simulink model "THIPWM_Three_Phase_Two_Level_Inverter"  (R2022a)
settings: Solver=ode4  StartTime=0.0  StopTime=1  FixedStep=1e-5  RelTol=1e-3
libraries: spsIGBTLib x6, spsSeriesRLCBranchLib x3, spsDCVoltageSourceLib x1, spsGroundLib x1, spsSawtoothGeneratorLib x1, spsThreePhaseVIMeasurementLib x1, spspowerguiLib x1
settings Model: Creator=nikos  LastModifiedBy=nikos

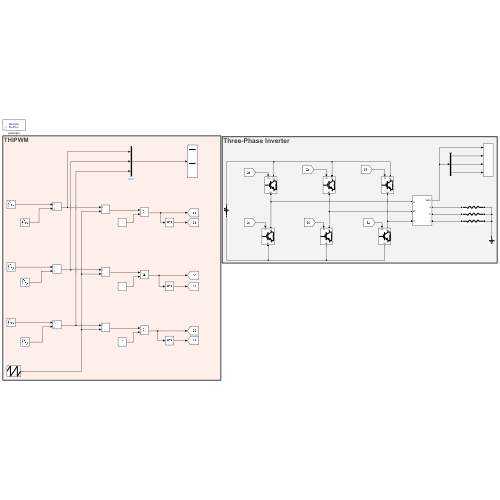
[thumbnail: Simulink's stored preview of the top-level diagram]
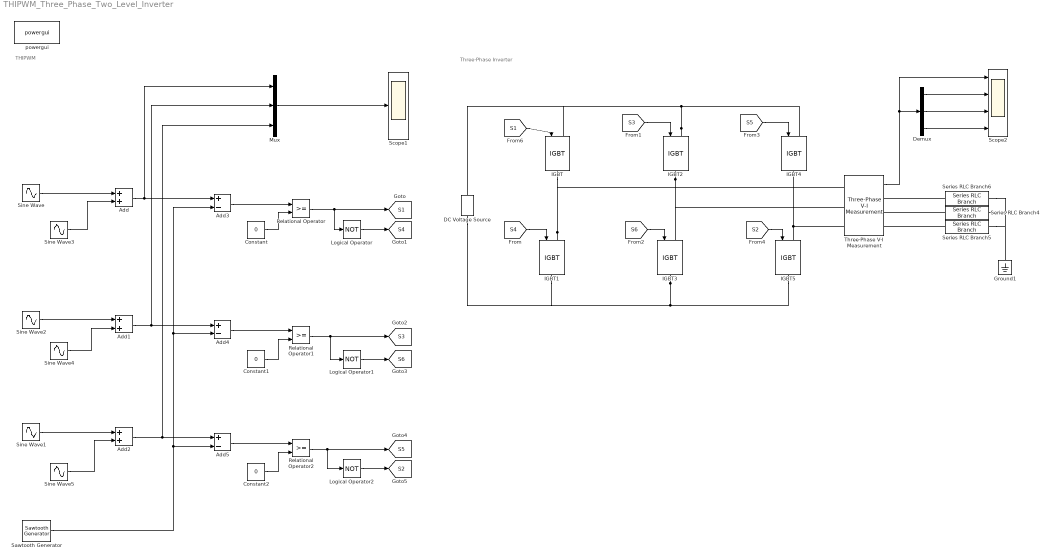
== system THIPWM_Three_Phase_Two_Level_Inverter ==
  note: THIPWM
  note: Three-Phase Inverter
  Add : Sum
  Add1 : Sum
  Add2 : Sum
  Add3 : Sum  Inputs=+-
  Add4 : Sum  Inputs=+-
  Add5 : Sum  Inputs=+-
  Constant : Constant  Value=0
  Constant1 : Constant  Value=0
  Constant2 : Constant  Value=0
  DC Voltage Source : spsDCVoltageSourceLib/DC Voltage Source  Amplitude=400  Measurements=None
  Demux : Demux  Outputs=3
  Ground1 : spsGroundLib/Ground  LConnTagsString=a
  IGBT{,1..5} (6 alike) : spsIGBTLib/IGBT  Ron=0.001  Lon=0  Vf=1  Tf=1e-6  Tt=2e-6  IC=0  Rs=1e5  Cs=inf  Measurements=off
  Logical Operator : Logic  Operator=NOT  AllPortsSameDT=off  OutDataTypeStr=boolean
  Logical Operator1 : Logic  Operator=NOT  AllPortsSameDT=off  OutDataTypeStr=boolean
  Logical Operator2 : Logic  Operator=NOT  AllPortsSameDT=off  OutDataTypeStr=boolean
  Mux : Mux  Inputs=3
  Relational Operator : RelationalOperator  OutDataTypeStr=boolean  RndMeth=Simplest  InputSameDT=off
  Relational Operator1 : RelationalOperator  OutDataTypeStr=boolean  RndMeth=Simplest  InputSameDT=off
  Relational Operator2 : RelationalOperator  OutDataTypeStr=boolean  RndMeth=Simplest  InputSameDT=off
  Sawtooth Generator : spsSawtoothGeneratorLib/Sawtooth Generator  Freq=2e3  Phase=180  Ts=0
  Scope1 : Scope
  Scope2 : Scope  NumInputPorts=4
  Series RLC Branch4 : spsSeriesRLCBranchLib/Series RLC Branch  LConnTagsString=__new0  RConnTagsString=__new0  BranchType=R  Resistance=100  Inductance=1e-3  SetiL0=off  InitialCurrent=0  Capacitance=1e-6  Setx0=off  InitialVoltage=0  Measurements=None
  Series RLC Branch5 : spsSeriesRLCBranchLib/Series RLC Branch  LConnTagsString=__new0  RConnTagsString=__new0  BranchType=R  Resistance=100  Inductance=1e-3  SetiL0=off  InitialCurrent=0  Capacitance=1e-6  Setx0=off  InitialVoltage=0  Measurements=None
  Series RLC Branch6 : spsSeriesRLCBranchLib/Series RLC Branch  LConnTagsString=__new0  RConnTagsString=__new0  BranchType=R  Resistance=100  Inductance=1e-3  SetiL0=off  InitialCurrent=0  Capacitance=1e-6  Setx0=off  InitialVoltage=0  Measurements=None
  Sine Wave : Sin  Amplitude=1.1547  Frequency=2*pi*50  SampleTime=0
  Sine Wave1 : Sin  Amplitude=1.1547  Frequency=2*pi*50  Phase=4*pi/3  SampleTime=0
  Sine Wave2 : Sin  Amplitude=1.1547  Frequency=2*pi*50  Phase=2*pi/3  SampleTime=0
  Sine Wave3 : Sin  Amplitude=0.193  Frequency=2*pi*50*3  SampleTime=0
  Sine Wave4 : Sin  Amplitude=0.193  Frequency=2*pi*50*3  SampleTime=0
  Sine Wave5 : Sin  Amplitude=0.193  Frequency=2*pi*50*3  SampleTime=0
  Three-Phase V-I Measurement : spsThreePhaseVIMeasurementLib/Three-Phase V-I Measurement  VoltageMeasurement=phase-to-ground  SetLabelV=off  LabelV=Vabc  Vpu=off  VpuLL=off  CurrentMeasurement=no  SetLabelI=off  LabelI=Iabc  Ipu=off  Pbase=100e6  Vbase=500e3  OutputType=Complex  PhasorSimulation=off  PSBequivalent=0
  powergui : spspowerguiLib/powergui  Priority=1  SimulationMode=Discrete  SampleTime=50e-6  frequency=60  Iterations=50  frequencyindice=0  Pbase=100e6  ErrMax=1e-4  UnitsV=kV  UnitsW=MW  buscounter=0  FunctionMessages=off  echomessages=off  EnableUseOfTLC=off  CurrentSourceSwitches=off  DisableSnubberDevices=off  DisableRonSwitches=off  DisableVfSwitches=off  DisplayEquations=off  AutomaticDiscreteSolvers=off  SolverType=Tustin/Backward Euler (TBE)  Interpol=off  ExternalGateDelay=off  methode=off  Ts=100  x0status=blocks  SPID=on  SwTol=0  HookPort=off  NonlinearTolerance=1e-4  nMaxIteration=100  ContinueOnMaxIteration=off  RestoreLinks=warning  ResistiveCurrentMeasurement=off  Frange=[0:2:500]  Ylog=off  Xlog=on  ShowGrid=off  save=off  variable=ZData  structure=0  ZoomFFT=off  StartTime=0.0  cycles=1  DisplayStyle=1  fundamental=60  FreqAxis=off  MaxFrequency=1000  frequencyindicesteady=1  RmsSteady=1  display=off
  tag scope: S1=global, S2=global, S3=global, S4=global, S5=global, S6=global
  wires:
  Sine Wave/1 -> Add/1
  Sine Wave3/1 -> Add/2
  Sine Wave2/1 -> Add1/1
  Sine Wave4/1 -> Add1/2
  Sine Wave1/1 -> Add2/1
  Sine Wave5/1 -> Add2/2
  Add/1 -> Mux/1, Add3/1
  Sawtooth Generator/1 -> Add5/2, Add4/2, Add3/2
  Add2/1 -> Mux/3, Add5/1
  Add1/1 -> Add4/1, Mux/2
  Add3/1 -> Relational Operator/1
  Add4/1 -> Relational Operator1/1
  Add5/1 -> Relational Operator2/1
  Constant/1 -> Relational Operator/2
  Constant1/1 -> Relational Operator1/2
  Constant2/1 -> Relational Operator2/2
  Relational Operator/1 -> Logical Operator/1, [S1]
  Logical Operator/1 -> [S4]
  Relational Operator1/1 -> Logical Operator1/1, [S3]
  Logical Operator1/1 -> [S6]
  Relational Operator2/1 -> Logical Operator2/1, [S5]
  Logical Operator2/1 -> [S2]
  [S3] -> IGBT2/1
  [S6] -> IGBT3/1
  Demux/1 -> Scope2/2
  Demux/2 -> Scope2/3
  [S5] -> IGBT4/1
  [S2] -> IGBT5/1
  Three-Phase V-I Measurement/1 -> Demux/1, Scope2/1
  [S4] -> IGBT1/1
  [S1] -> IGBT/1
  Demux/3 -> Scope2/4
  Mux/1 -> Scope1/1
  connections:
  Series RLC Branch4/LConn1 -- Ground1/LConn1 -- Series RLC Branch5/LConn1 -- Series RLC Branch6/LConn1
  IGBT1/LConn1 -- IGBT/RConn1 -- Three-Phase V-I Measurement/LConn1
  Three-Phase V-I Measurement/LConn3 -- IGBT5/LConn1 -- IGBT4/RConn1
  IGBT2/RConn1 -- IGBT3/LConn1 -- Three-Phase V-I Measurement/LConn2
  IGBT3/RConn1 -- DC Voltage Source/LConn1 -- IGBT1/RConn1 -- IGBT5/RConn1
  IGBT2/LConn1 -- IGBT4/LConn1 -- DC Voltage Source/RConn1 -- IGBT/LConn1
  Series RLC Branch5/RConn1 -- Three-Phase V-I Measurement/RConn3
  Series RLC Branch6/RConn1 -- Three-Phase V-I Measurement/RConn1
  Series RLC Branch4/RConn1 -- Three-Phase V-I Measurement/RConn2
